simulink model "gantrycrane_animation"  (Simulink 8.3)
settings: Solver=ode45  StartTime=0.0  StopTime=50  RelTol=1e-3
undefined symbols (not defined in the file or in its folder): drawGantryCrane
settings Model: Creator=nedward  LastModifiedBy=jhl48
settings OptimizationCC: ExpressionDepthLimit=2147483647
settings DebuggingCC: FcnCallInpInsideContextMsg=UseLocalSettings

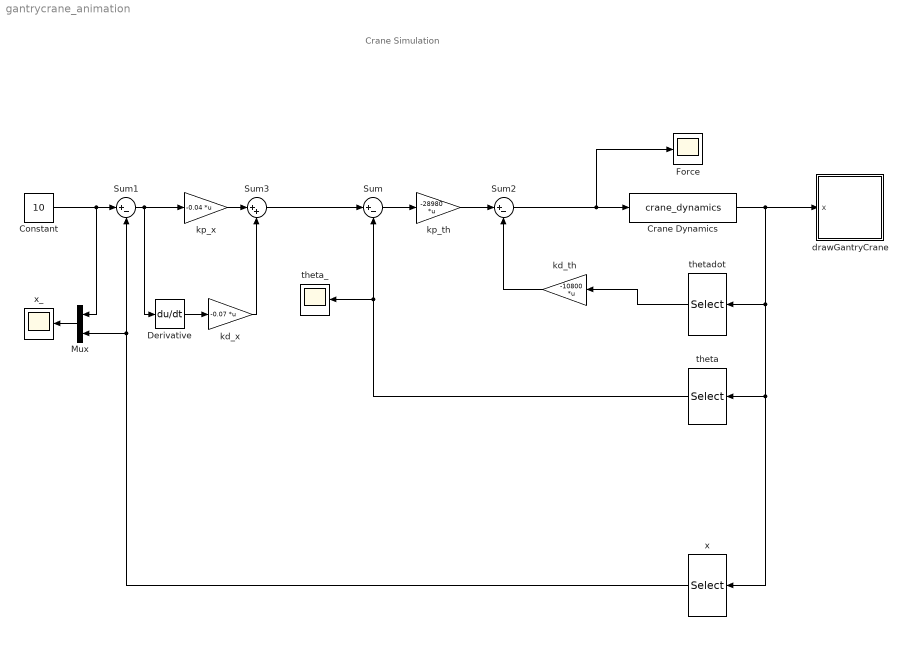
== system gantrycrane_animation ==
  note: Crane Simulation
  Constant : Constant  Value=10
  Crane Dynamics : S-Function  FunctionName=crane_dynamics  Parameters=P  EnableBusSupport=off
  Derivative : Derivative
  Force : Scope
      settings: TimeRange=50  YMin=-5000  YMax=20000
  Mux : Mux  Inputs=2
  Sum : Sum  Inputs=|+-
  Sum1 : Sum  Inputs=|+-
  Sum2 : Sum  Inputs=|+-
  Sum3 : Sum  Inputs=|++
  drawGantryCrane : Subsystem
      mask init:
      | bar = 20;
      | crane = [5 3];
      | L1 = 6;
      | R1 = 1;
      | L2 = 15;
      | R2 = 0.5;
      mask Display: image(imread('tv.jpg'))
  kd_th : Gain  Gain=-10800  Multiplication=Matrix(K*u)
  kd_x : Gain  Gain=-0.07  Multiplication=Matrix(K*u)
  kp_th : Gain  Gain=-28980  Multiplication=Matrix(K*u)
  kp_x : Gain  Gain=-0.04  Multiplication=Matrix(K*u)
  theta : Selector  InputPortWidth=6  Indices=[5]
  theta_ : Scope
      settings: TimeRange=50  YMin=-0.25  YMax=0.3
  thetadot : Selector  InputPortWidth=6  Indices=[2]
  x : Selector  InputPortWidth=6  Indices=[4]
  x_ : Scope
      settings: TimeRange=50  YMin=0  YMax=12.5  SaveName=ScopeData2
  wires:
  Crane Dynamics/1 -> drawGantryCrane/1(x), theta/1, x/1, thetadot/1
  Sum/1 -> kp_th/1
  theta/1 -> Sum/2, theta_/1
  x/1 -> Mux/2, Sum1/2
  thetadot/1 -> kd_th/1
  Sum1/1 -> Derivative/1, kp_x/1
  Sum3/1 -> Sum/1
  kd_th/1 -> Sum2/2
  Sum2/1 -> Crane Dynamics/1, Force/1
  kp_th/1 -> Sum2/1
  Mux/1 -> x_/1
  kp_x/1 -> Sum3/1
  kd_x/1 -> Sum3/2
  Derivative/1 -> kd_x/1
  Constant/1 -> Mux/1, Sum1/1

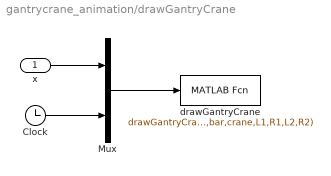
== system gantrycrane_animation/drawGantryCrane ==
  x : Inport
  Clock : Clock
  Mux : Mux  Inputs=2
  drawGantryCrane : MATLABFcn  MATLABFcn=drawGantryCrane(u,bar,crane,L1,R1,L2,R2)  OutputDimensions=0  SampleTime=0.01
  wires:
  Mux/1 -> drawGantryCrane/1
  x/1 -> Mux/1
  Clock/1 -> Mux/2
